simulink model "mdl_control_pd_16b"  (R2016b)
settings: Solver=FixedStepDiscrete  StartTime=0.0  StopTime=20  FixedStep=0.001  RelTol=1e-3
undefined symbols (not defined in the file or in its folder): Par_control_pd
settings Model: Creator=Nu  LastModifiedBy=Nu

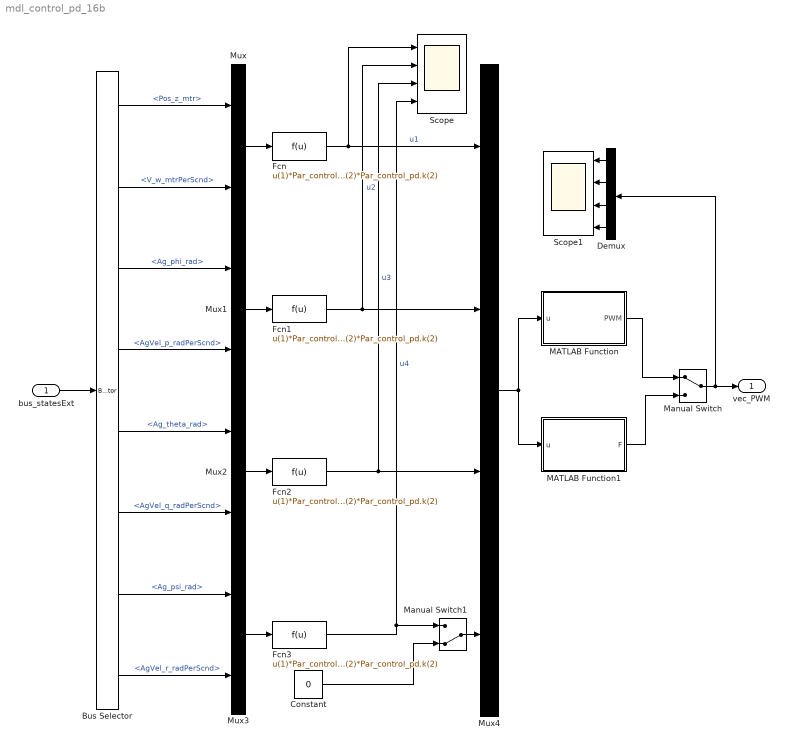
== system mdl_control_pd_16b ==
  bus_statesExt : Inport  OutDataTypeStr=Bus: mdl_statesExt
  Bus Selector : BusSelector  OutputSignals=Pos_z_mtr,V_w_mtrPerScnd,Ag_phi_rad,AgVel_p_radPerScnd,Ag_theta_rad,AgVel_q_radPerScnd,Ag_psi_rad,AgVel_r_radPerScnd
  Constant : Constant  Value=0
  Demux : Demux
  Fcn{,1..3} (4 alike) : Fcn  Expr=u(1)*Par_control_pd.k(1) + u(2)*Par_control_pd.k(2)
  MATLAB Function : MATLAB Function  TreatAsAtomicUnit=on
  MATLAB Function1 : MATLAB Function  TreatAsAtomicUnit=on
  Manual Switch : ManualSwitch
  Manual Switch1 : ManualSwitch  CurrentSetting=0
  Mux{,1..3} (4 alike) : Mux  Inputs=2
  Mux4 : Mux
  Scope : Scope  NumInputPorts=4
  Scope1 : Scope  NumInputPorts=4
  "vec_PWM " : Outport
  wires:
  MATLAB Function/1(PWM) -> Manual Switch/1
  Constant/1 -> Manual Switch1/2
  Bus Selector/8 -> Mux3/2  "<AgVel_r_radPerScnd>"
  Bus Selector/7 -> Mux3/1  "<Ag_psi_rad>"
  Bus Selector/6 -> Mux2/2  "<AgVel_q_radPerScnd>"
  Bus Selector/5 -> Mux2/1  "<Ag_theta_rad>"
  Bus Selector/4 -> Mux1/2  "<AgVel_p_radPerScnd>"
  Bus Selector/3 -> Mux1/1  "<Ag_phi_rad>"
  Bus Selector/2 -> Mux/2  "<V_w_mtrPerScnd>"
  Bus Selector/1 -> Mux/1  "<Pos_z_mtr>"
  bus_statesExt/1 -> Bus Selector/1
  Demux/4 -> Scope1/4
  Demux/3 -> Scope1/3
  Demux/2 -> Scope1/2
  Demux/1 -> Scope1/1
  Mux4/1 -> MATLAB Function1/1(u), MATLAB Function/1(u)
  Fcn3/1 -> Manual Switch1/1, Scope/4  "u4"
  Fcn2/1 -> Mux4/3, Scope/3  "u3"
  Fcn1/1 -> Scope/2, Mux4/2  "u2"
  Fcn/1 -> Mux4/1, Scope/1  "u1"
  Mux3/1 -> Fcn3/1
  Mux1/1 -> Fcn1/1
  Mux2/1 -> Fcn2/1
  Mux/1 -> Fcn/1
  Manual Switch/1 -> "vec_PWM "/1, Demux/1
  MATLAB Function1/1(F) -> Manual Switch/2
  Manual Switch1/1 -> Mux4/4

== matlab function mdl_control_pd_16b/MATLAB Function ==
  data: u input; PWM output; Par_mdlQuad parameter
function PWM = fcn(u, Par_mdlQuad)

pwm = Par_mdlQuad.ca_esc^-1 * u;
PWM = pwm + Par_mdlQuad.PWM0;

== matlab function mdl_control_pd_16b/MATLAB Function1 ==
  data: u input; F output; Par_mdlQuad parameter
function F = fcn(u, Par_mdlQuad)

f = Par_mdlQuad.ca^-1 * u;
F = f + Par_mdlQuad.F0;
